simulink model "ex3_triggered"  (R2021a)
settings: Solver=FixedStepAuto  StartTime=0.0  StopTime=10.0  FixedStep=1e-3  RelTol=1e-3
settings Model: Creator=reemb  LastModifiedBy=reemb

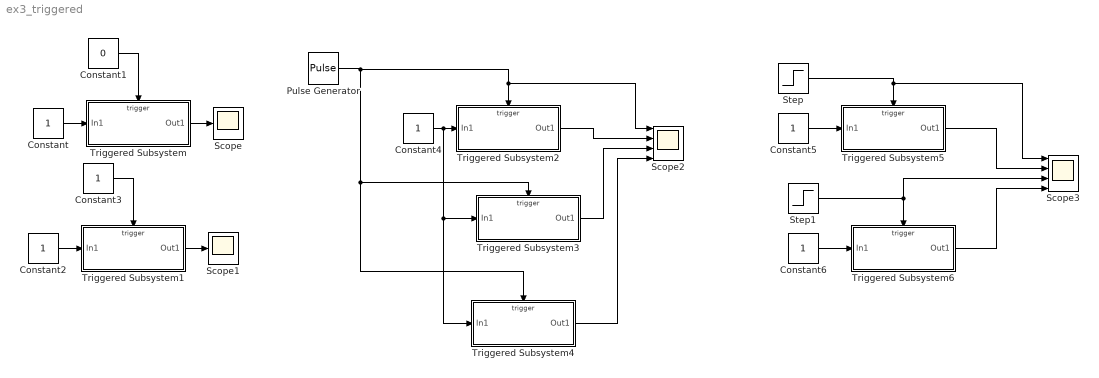
== system ex3_triggered ==
  Constant{,2..6} (6 alike) : Constant
  Constant1 : Constant  Value=0
  Pulse Generator : DiscretePulseGenerator  PulseType=Time based  PulseWidth=50
  Scope : Scope
  Scope1 : Scope
  Scope2 : Scope  NumInputPorts=4
  Scope3 : Scope  NumInputPorts=4
  Step : Step  Before=-1  After=0  SampleTime=0
  Step1 : Step  Before=2  After=0  SampleTime=0
  Triggered Subsystem : Subsystem  TreatAsAtomicUnit=on
  Triggered Subsystem1 : Subsystem  TreatAsAtomicUnit=on
  Triggered Subsystem2 : Subsystem  TreatAsAtomicUnit=on
  Triggered Subsystem3 : Subsystem  TreatAsAtomicUnit=on
  Triggered Subsystem4 : Subsystem  TreatAsAtomicUnit=on
  Triggered Subsystem5 : Subsystem  TreatAsAtomicUnit=on
  Triggered Subsystem6 : Subsystem  TreatAsAtomicUnit=on
  wires:
  Constant/1 -> Triggered Subsystem/1(In1)
  Triggered Subsystem/1(Out1) -> Scope/1
  Constant1/1 -> Triggered Subsystem/Trigger
  Constant3/1 -> Triggered Subsystem1/Trigger
  Triggered Subsystem1/1(Out1) -> Scope1/1
  Constant2/1 -> Triggered Subsystem1/1(In1)
  Triggered Subsystem2/1(Out1) -> Scope2/2
  Pulse Generator/1 -> Triggered Subsystem4/Trigger, Triggered Subsystem3/Trigger, Scope2/1, Triggered Subsystem2/Trigger
  Triggered Subsystem3/1(Out1) -> Scope2/3
  Constant4/1 -> Triggered Subsystem4/1(In1), Triggered Subsystem3/1(In1), Triggered Subsystem2/1(In1)
  Triggered Subsystem4/1(Out1) -> Scope2/4
  Constant5/1 -> Triggered Subsystem5/1(In1)
  Triggered Subsystem5/1(Out1) -> Scope3/2
  Step/1 -> Triggered Subsystem5/Trigger, Scope3/1
  Step1/1 -> Scope3/3, Triggered Subsystem6/Trigger
  Constant6/1 -> Triggered Subsystem6/1(In1)
  Triggered Subsystem6/1(Out1) -> Scope3/4

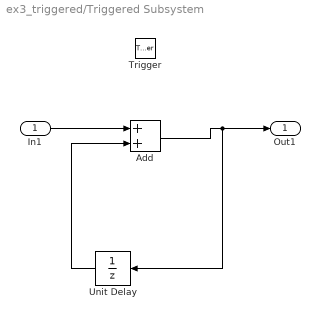
== system ex3_triggered/Triggered Subsystem ==
  In1 : Inport
  Trigger : TriggerPort  VariantControl=(inherit)
  Add : Sum
  Unit Delay : UnitDelay  SampleTime=-1  HasFrameUpgradeWarning=on
  Out1 : Outport
  wires:
  In1/1 -> Add/1
  Add/1 -> Unit Delay/1, Out1/1
  Unit Delay/1 -> Add/2

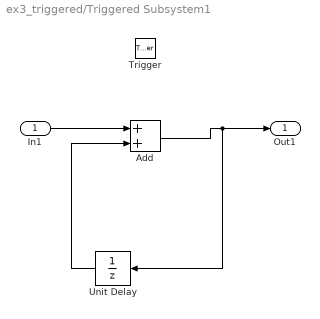
== system ex3_triggered/Triggered Subsystem1 ==
  In1 : Inport
  Trigger : TriggerPort  VariantControl=(inherit)
  Add : Sum
  Unit Delay : UnitDelay  SampleTime=-1  HasFrameUpgradeWarning=on
  Out1 : Outport
  wires:
  Unit Delay/1 -> Add/2
  Add/1 -> Out1/1, Unit Delay/1
  In1/1 -> Add/1

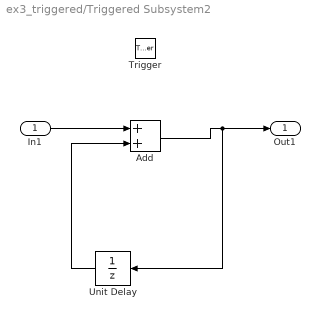
== system ex3_triggered/Triggered Subsystem2 ==
  In1 : Inport
  Trigger : TriggerPort  VariantControl=(inherit)
  Add : Sum
  Unit Delay : UnitDelay  SampleTime=-1  HasFrameUpgradeWarning=on
  Out1 : Outport
  wires:
  In1/1 -> Add/1
  Add/1 -> Unit Delay/1, Out1/1
  Unit Delay/1 -> Add/2

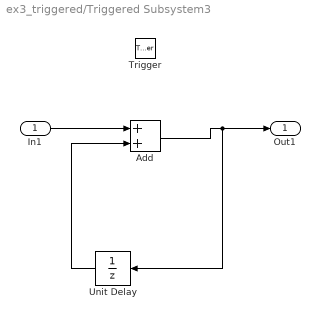
== system ex3_triggered/Triggered Subsystem3 ==
  In1 : Inport
  Trigger : TriggerPort  TriggerType=falling  VariantControl=(inherit)
  Add : Sum
  Unit Delay : UnitDelay  SampleTime=-1  HasFrameUpgradeWarning=on
  Out1 : Outport
  wires:
  Unit Delay/1 -> Add/2
  Add/1 -> Out1/1, Unit Delay/1
  In1/1 -> Add/1

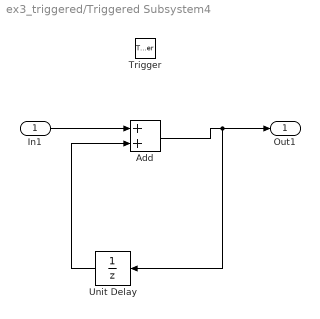
== system ex3_triggered/Triggered Subsystem4 ==
  In1 : Inport
  Trigger : TriggerPort  TriggerType=either  VariantControl=(inherit)
  Add : Sum
  Unit Delay : UnitDelay  SampleTime=-1  HasFrameUpgradeWarning=on
  Out1 : Outport
  wires:
  In1/1 -> Add/1
  Add/1 -> Unit Delay/1, Out1/1
  Unit Delay/1 -> Add/2

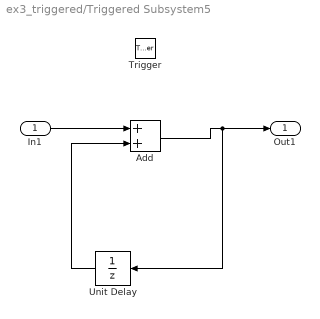
== system ex3_triggered/Triggered Subsystem5 ==
  In1 : Inport
  Trigger : TriggerPort  VariantControl=(inherit)
  Add : Sum
  Unit Delay : UnitDelay  SampleTime=-1  HasFrameUpgradeWarning=on
  Out1 : Outport
  wires:
  Unit Delay/1 -> Add/2
  Add/1 -> Out1/1, Unit Delay/1
  In1/1 -> Add/1

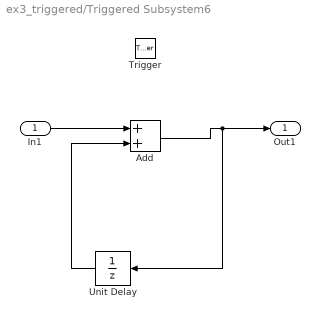
== system ex3_triggered/Triggered Subsystem6 ==
  In1 : Inport
  Trigger : TriggerPort  TriggerType=falling  VariantControl=(inherit)
  Add : Sum
  Unit Delay : UnitDelay  SampleTime=-1  HasFrameUpgradeWarning=on
  Out1 : Outport
  wires:
  In1/1 -> Add/1
  Add/1 -> Unit Delay/1, Out1/1
  Unit Delay/1 -> Add/2
